simulink model "modelPID"  (Simulink 8.2)
settings: Solver=ode4  StartTime=0.0  StopTime=TKoniec  FixedStep=T0  RelTol=1e-3
values from neighbouring files (symbols this model uses):
  D = input(3)    [opt_pid.m]    (also in parametryPID.m = 1.38)
  I = Nastawy(2)    [LP1.m]    (also in USImodel.m; opt_pid.m = input(2); parametryPID.m = 0.88; wskaJak1.m = params(2))
  P = Nastawy(1)    [LP1.m]    (also in USImodel.m; opt_pid.m = input(1); parametryPID.m = 1.5; wskaJak1.m = params(1))
undefined symbols (not defined in the file or in its folder): a, fv, Hv_odwr, Iv, Jv, lv, magnitude, Thrust
libraries: simulink_need_slupdate x1
settings Model: Creator=Michal  LastModifiedBy=Aga
settings OptimizationCC: ExpressionDepthLimit=128
settings DebuggingCC: MultiTaskDSMMsg=warning  MultiTaskCondExecSysMsg=none  FcnCallInpInsideContextMsg=EnableAllAsWarning  StateNameClashWarn=none
settings RTWCC: IncludeERTFirstTime=on

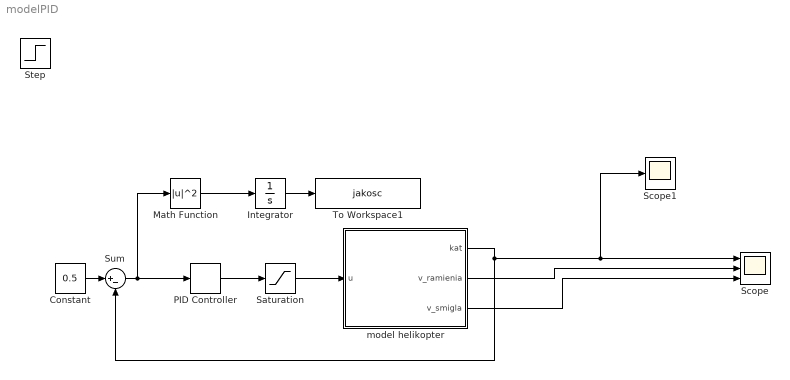
== system modelPID ==
  Constant : Constant  Value=0.5
  Integrator : Integrator
  Math Function : Math  Operator=magnitude^2  SaturateOnIntegerOverflow=on
  PID Controller : simulink_need_slupdate/PID Controller  P=P  I=I  D=D
  Saturation : Saturate  UpperLimit=1  LowerLimit=-1
  Scope : Scope  NumInputPorts=3
      settings: YMin=-5~-5~-5  YMax=5~5~5
  Scope1 : Scope
  Step : Step  SampleTime=0
  Sum : Sum  Inputs=|+-
  To Workspace1 : ToWorkspace  VariableName=jakosc  SampleTime=-1
  "model helikopter " : Subsystem
  wires:
  PID Controller/1 -> Saturation/1
  Sum/1 -> Math Function/1, PID Controller/1
  Integrator/1 -> To Workspace1/1
  "model helikopter "/1(kat) -> Scope1/1, Scope/1, Sum/2
  Saturation/1 -> "model helikopter "/1(u)
  Math Function/1 -> Integrator/1
  "model helikopter "/2(v_ramienia) -> Scope/2
  "model helikopter "/3(v_smigla) -> Scope/3
  Constant/1 -> Sum/1

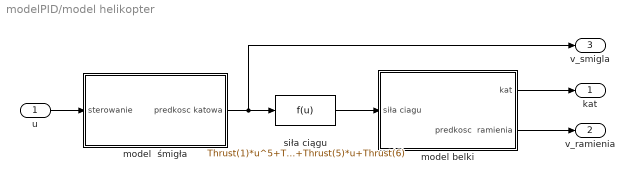
== system modelPID/model helikopter  ==
  u : Inport
  model  śmigła : Subsystem
  model belki : Subsystem
  siła ciągu : Fcn  Expr=Thrust(1)*u^5+Thrust(2)*u^4+Thrust(3)*u^3+Thrust(4)*u^2+Thrust(5)*u+Thrust(6)
  kat : Outport
  v_ramienia : Outport  Port=2
  v_smigla : Outport  Port=3
  wires:
  model  śmigła/1(predkosc katowa) -> v_smigla/1, siła ciągu/1
  u/1 -> model  śmigła/1(sterowanie)
  siła ciągu/1 -> model belki/1("siła ciagu ")
  model belki/1(kat) -> kat/1
  model belki/2(predkosc  ramienia) -> v_ramienia/1

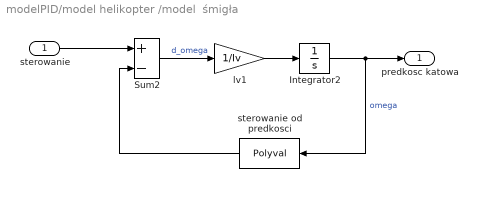
== system modelPID/model helikopter /model  śmigła ==
  sterowanie : Inport
  Integrator2 : Integrator
  Sum2 : Sum  Inputs=+-
  lv1 : Gain  Gain=1/Iv
  sterowanie od predkosci : Polyval  Coefs=Hv_odwr
  predkosc katowa : Outport
  wires:
  Integrator2/1 -> predkosc katowa/1, sterowanie od predkosci/1  "omega"
  lv1/1 -> Integrator2/1
  Sum2/1 -> lv1/1  "d_omega"
  sterowanie od predkosci/1 -> Sum2/2
  sterowanie/1 -> Sum2/1

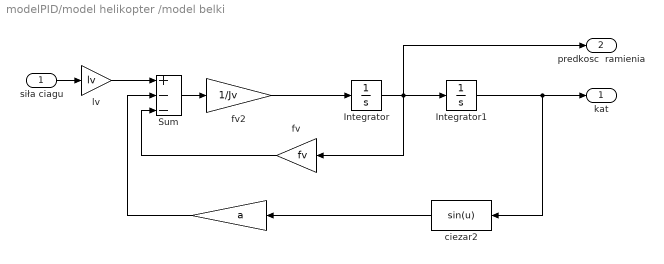
== system modelPID/model helikopter /model belki ==
  "siła ciagu " : Inport
  "  " : Gain  Gain=a
  Integrator : Integrator
  Integrator1 : Integrator
  Sum : Sum  Inputs=+--
  ciezar2 : Fcn  Expr=sin(u)
  fv : Gain  Gain=fv
  fv2 : Gain  Gain=1/Jv
  lv : Gain  Gain=lv
  kat : Outport
  predkosc  ramienia : Outport  Port=2
  wires:
  "siła ciagu "/1 -> lv/1
  Sum/1 -> fv2/1
  Integrator/1 -> predkosc  ramienia/1, fv/1, Integrator1/1
  "  "/1 -> Sum/2
  fv/1 -> Sum/3
  Integrator1/1 -> kat/1, ciezar2/1
  fv2/1 -> Integrator/1
  ciezar2/1 -> "  "/1
  lv/1 -> Sum/1
